simulink subsystem "Engineering_to_Actuator"  (R2024a)
settings: Solver=VariableStepAuto  StartTime=0.0  StopTime=10.0  RelTol=1e-3
undefined symbols (not defined in the file or in its folder): vehicle
settings Model: Creator=gurt1  LastModifiedBy=gurt1

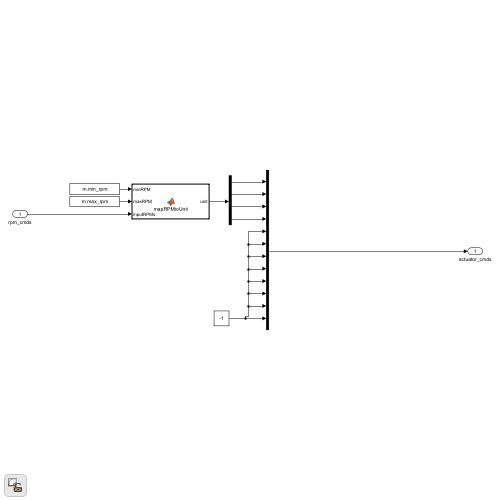
[thumbnail: Simulink's stored preview of the top-level diagram]
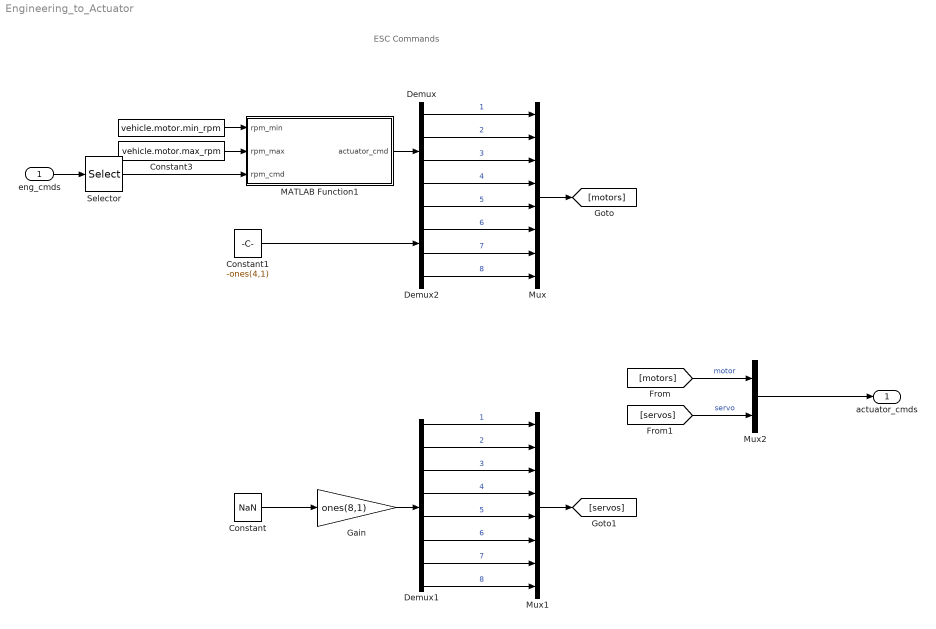
== system Engineering_to_Actuator ==
  note: ESC Commands
  eng_cmds : Inport
  " " : Constant  Value=vehicle.motor.min_rpm
  Constant : Constant  Value=NaN
  Constant1 : Constant  Value=-ones(4,1)
  Constant3 : Constant  Value=vehicle.motor.max_rpm
  Demux : Demux
  Demux1 : Demux  Outputs=8
  Demux2 : Demux
  Gain : Gain  Gain=ones(8,1)
  MATLAB Function1 : MATLAB Function  TreatAsAtomicUnit=on
  Mux : Mux  Inputs=8
  Mux1 : Mux  Inputs=8
  Mux2 : Mux  Inputs=2
  Selector : Selector  InputPortWidth=16  IndexOptions=Index vector (dialog)  Indices=[1:4]  OutputSizes=1
  actuator_cmds : Outport
  wires:
  Demux/4 -> Mux/4  "4"
  Demux/1 -> Mux/1  "1"
  Constant3/1 -> MATLAB Function1/2(rpm_max)
  Demux/2 -> Mux/2  "2"
  " "/1 -> MATLAB Function1/1(rpm_min)
  MATLAB Function1/1(actuator_cmd) -> Demux/1
  Demux/3 -> Mux/3  "3"
  eng_cmds/1 -> Selector/1
  Constant/1 -> Gain/1
  Gain/1 -> Demux1/1
  Demux2/1 -> Mux/5  "5"
  Demux2/2 -> Mux/6  "6"
  Demux2/3 -> Mux/7  "7"
  Demux2/4 -> Mux/8  "8"
  Mux/1 -> [motors]
  Demux1/1 -> Mux1/1  "1"
  Demux1/2 -> Mux1/2  "2"
  Demux1/3 -> Mux1/3  "3"
  Demux1/4 -> Mux1/4  "4"
  Demux1/5 -> Mux1/5  "5"
  Demux1/6 -> Mux1/6  "6"
  Demux1/7 -> Mux1/7  "7"
  Demux1/8 -> Mux1/8  "8"
  Mux1/1 -> [servos]
  Mux2/1 -> actuator_cmds/1
  [motors] -> Mux2/1  "motor"
  [servos] -> Mux2/2  "servo"
  Selector/1 -> MATLAB Function1/3(rpm_cmd)
  Constant1/1 -> Demux2/1

== matlab function Engineering_to_Actuator/MATLAB Function1 ==
  data: rpm_min input; actuator_cmd output; rpm_max input; rpm_cmd input
function actuator_cmd = map_rpm_to_actuator(rpm_min, rpm_max, rpm_cmd)

actuator_cmd = map_rpm_to_actuator(rpm_min, rpm_max, rpm_cmd);
